simulink model "quadrotorbacksteppingsimulationtracker"  (R2015a)
settings: Solver=ode45  StartTime=0.0  StopTime=15  FixedStep=1e-3  RelTol=1e-3
settings Model: Creator=kbmaj  LastModifiedBy=kbmaj

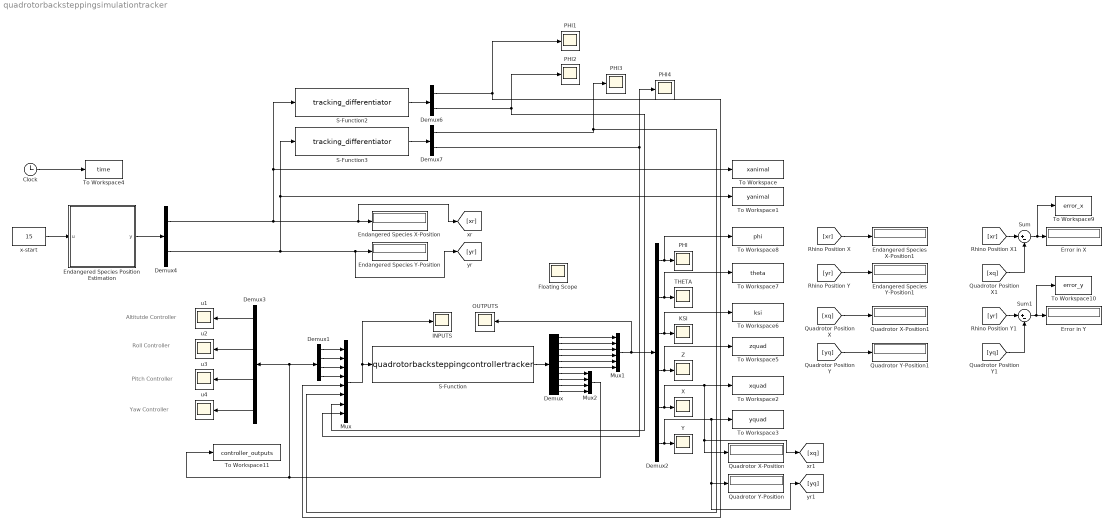
== system quadrotorbacksteppingsimulationtracker ==
  note: Yaw Controller
  note: Pitch Controller
  note: Roll Controller
  note: Altitutde Controller
  Clock : Clock
  Demux : Demux  Outputs=10
  Demux1 : Demux
  Demux2 : Demux  Outputs=6
  Demux3 : Demux
  Demux4 : Demux  Outputs=2
  Demux6 : Demux  Outputs=2
  Demux7 : Demux  Outputs=2
  Endangered Species Position Estimation : MATLAB Function  TreatAsAtomicUnit=on
  Endangered Species X-Position : Display
  Endangered Species X-Position1 : Display
  Endangered Species Y-Position : Display
  Endangered Species Y-Position1 : Display
  Error in X : Display
  Error in Y : Display
  Floating Scope : Scope
      settings: Floating=on  YMin=-30  YMax=45  SaveName=ScopeData12
  INPUTS : Scope
      settings: YMin=-10000  YMax=150000
  KSI : Scope
      settings: YMin=-1359.25  YMax=-1354.25  SaveName=ScopeData4
  Mux : Mux  Inputs=8
  Mux1 : Mux  Inputs=6
  Mux2 : Mux
  OUTPUTS : Scope
      settings: YMin=-10000  YMax=150000  SaveName=ScopeData11
  PHI{,1..4} (5 alike) : Scope
      PHI settings: TimeRange=10  YMin=1250  YMax=3750  SaveName=ScopeData2
      PHI1 settings: TimeRange=10  YMin=9.75  YMax=12.75  SaveName=ScopeData13
      PHI2 settings: TimeRange=10  YMin=1250  YMax=3750  SaveName=ScopeData14
      PHI3 settings: TimeRange=10  YMin=1250  YMax=3750  SaveName=ScopeData15
      PHI4 settings: TimeRange=10  YMin=1250  YMax=3750  SaveName=ScopeData16
  Quadrotor X-Position : Display
  Quadrotor X-Position1 : Display
  Quadrotor Y-Position : Display
  Quadrotor Y-Position1 : Display
  S-Function : S-Function  FunctionName=quadrotorbacksteppingcontrollertracker
  S-Function2 : S-Function  FunctionName=tracking_differentiator
  S-Function3 : S-Function  FunctionName=tracking_differentiator
  Sum : Sum  Inputs=|+-
  Sum1 : Sum  Inputs=|+-
  THETA : Scope
      settings: YMin=19  YMax=21  SaveName=ScopeData3
  To Workspace : ToWorkspace  VariableName=xanimal  SampleTime=-1
  To Workspace1 : ToWorkspace  VariableName=yanimal  SampleTime=-1
  To Workspace10 : ToWorkspace  VariableName=error_y  SampleTime=-1
  To Workspace11 : ToWorkspace  VariableName=controller_outputs  SampleTime=-1
  To Workspace2 : ToWorkspace  VariableName=xquad  SampleTime=-1
  To Workspace3 : ToWorkspace  VariableName=yquad  SampleTime=-1
  To Workspace4 : ToWorkspace  VariableName=time  SampleTime=-1
  To Workspace5 : ToWorkspace  VariableName=zquad  SampleTime=-1
  To Workspace6 : ToWorkspace  VariableName=ksi  SampleTime=-1
  To Workspace7 : ToWorkspace  VariableName=theta  SampleTime=-1
  To Workspace8 : ToWorkspace  VariableName=phi  SampleTime=-1
  To Workspace9 : ToWorkspace  VariableName=error_x  SampleTime=-1
  X : Scope
      settings: TimeRange=5  YMin=7.05  YMax=7.6  SaveName=ScopeData6
  Y : Scope
      settings: YMin=-60  YMax=60  SaveName=ScopeData7
  Z : Scope
      settings: YMin=9350  YMax=9465  SaveName=ScopeData5
  u{1..4} (4 alike) : Scope
      u1 settings: YMin=0  YMax=120000  SaveName=ScopeData8
      u2 settings: TimeRange=25  YMin=-0.2  YMax=0.5
      u3 settings: YMin=0  YMax=120000  SaveName=ScopeData10
      u4 settings: YMin=0  YMax=120000  SaveName=ScopeData9
  x-start : Constant  Value=15
  wires:
  S-Function/1 -> Demux/1
  Mux/1 -> INPUTS/1, S-Function/1
  Demux/1 -> Mux1/1
  Demux/2 -> Mux1/2
  Demux/3 -> Mux1/3
  Demux/4 -> Mux1/4
  Demux/5 -> Mux1/5
  Demux/6 -> Mux1/6
  Mux1/1 -> OUTPUTS/1, Demux2/1
  Demux2/1 -> To Workspace8/1, PHI/1
  Demux2/2 -> To Workspace7/1, THETA/1
  Demux2/3 -> To Workspace6/1, KSI/1
  Demux2/4 -> To Workspace5/1, Z/1
  Demux2/5 -> To Workspace2/1, [xq], Quadrotor X-Position/1, X/1
  Demux/7 -> Mux2/1
  Demux/8 -> Mux2/2
  Demux/9 -> Mux2/3
  Demux/10 -> Mux2/4
  Demux1/1 -> Mux/1
  Demux1/2 -> Mux/2
  Demux1/3 -> Mux/3
  Demux1/4 -> Mux/4
  Mux2/1 -> Demux1/1, Demux3/1, To Workspace11/1
  Demux3/1 -> u1/1
  Demux3/2 -> u2/1
  Demux3/3 -> u3/1
  Demux3/4 -> u4/1
  x-start/1 -> Endangered Species Position Estimation/1(u)
  Demux4/1 -> [xr], Endangered Species X-Position/1, S-Function2/1, To Workspace/1
  Demux4/2 -> [yr], Endangered Species Y-Position/1, S-Function3/1, To Workspace1/1
  Demux2/6 -> To Workspace3/1, [yq], Quadrotor Y-Position/1, Y/1
  Clock/1 -> To Workspace4/1
  Endangered Species Position Estimation/1(y) -> Demux4/1
  [xr] -> Endangered Species X-Position1/1
  [yr] -> Endangered Species Y-Position1/1
  [xq] -> Quadrotor X-Position1/1
  [yq] -> Quadrotor Y-Position1/1
  [xr] -> Sum/1
  [xq] -> Sum/2
  [yr] -> Sum1/1
  [yq] -> Sum1/2
  Sum1/1 -> To Workspace10/1, Error in Y/1
  Sum/1 -> To Workspace9/1, Error in X/1
  Demux6/1 -> Mux/5, PHI1/1
  Demux6/2 -> Mux/7, PHI2/1
  Demux7/1 -> PHI3/1, Mux/6
  Demux7/2 -> PHI4/1, Mux/8
  S-Function2/1 -> Demux6/1
  S-Function3/1 -> Demux7/1

== matlab function quadrotorbacksteppingsimulationtracker/Endangered Species Position Estimation ==
  data: y output; u input
function y = tracker(u)
%#codegen

% Initialization
B       = 1;  % distance between wheels
dt      = 1;  % sampling time
X       = 0;  % x-position of sensor
Y       = 0;  % y-position of sensor
v       = 1.5;        % velocity
%varphi  = 2.5*pi/80; % steering angle

% Noise Signals - q(k),r(k)
% Process(Q) and Observation(R) noise varainces, mean 0
mu          = 0;
sigma_x     = 0.05;
sigma_y     = 0.05;
sigma_phi   = pi/180;
sigma_r     = 0.5;
sigma_theta = 2*pi/180;

Q           = diag([sigma_x, sigma_y, sigma_phi].^2);
R           = diag([sigma_r, sigma_theta].^2);
p           = diag([0.0001 0.0001 0.000001]);

% System Initial States
x       = [ u ; -22; 0];
x_hat   = [ 15; -23; 0];

% Instance
kk = 50;
% Preallocation
 xestpos     = zeros(kk,1)';
 yestpos     = zeros(kk,1)';
% Discrete Dynamic Model

for k = 1:kk
% System Noises
qn          = [sigma_x*randn(1)+mu;  sigma_y*randn(1)+mu;  sigma_phi*randn(1)+mu]; % process noise
rn          = [sigma_r*randn(1)+mu;  sigma_theta*randn(1)+mu]; % measurement noise

% if k > 0 && k < 23
%         varphi  = 2.5*pi/80;
%     elseif k > 23 && k < 28
%         varphi = 0;
%     else if k >28 && k < 50
%         varphi = -2.5*pi/100;
%     end
% end

if k > 0 && k < 25;
varphi  =  2.5*pi/80;
else k > 25 && k <60;
varphi  = -2.5*pi/80;
end

% Model
% Perfect System Model - x(k+1)
x  =   x + [dt* v* cos(x(3)+varphi);
            dt* v* sin(x(3)+varphi);
            dt* (v/B) *(sin(varphi))];
x = x + qn;
% Perfect Output measurement
z    =       [sqrt((X-x(1))^2 + (Y-x(2))^2);
            atan(((Y-(x(2)))/(X-(x(1))))-((x(3))))];
Z = z + rn;
% EKF Model and Measurement
x_hat  = x_hat +  [dt* v* cos(x_hat(3)+varphi);
                   dt* v* sin(x_hat(3)+varphi);
                   dt* (v/B)*(sin(varphi))];
% Z measurement
Zh   = [sqrt((X-(x_hat(1)))^2 + (Y-x_hat(2))^2 );
       atan(((Y-(x_hat(2)))/((X-(x_hat(1)))))-((x_hat(3))))];

% F Model Jacobian
F_jac     =  [1 0  -dt*v*sin(x_hat(3) + varphi)
              0 1   dt*v*cos(x_hat(3) + varphi)
              0 0   1                         ];
% H Measurement Jacobian
d       = sqrt((X-x_hat(1))^2+(Y-x_hat(2))^2);
H_jac   = [(x_hat(1)-X)/d    (x_hat(2)-Y)/d      0
          -(x_hat(2)-Y)/d^2  (x_hat(1)-X)/d^2   -1];

% Prediction Function
p   =  F_jac * p * F_jac' + Q;

% Updates
S   =  H_jac * p       * H_jac' + R;
K   =  p     * H_jac'  * inv(S);

% Estimates
x_est = x_hat + K*(Z-Zh);
p_est = p - K*S*K';
%x_est;

xestpos(k) = x_est(1);
yestpos(k) = x_est(2);
xxx = x_est(1);
yyy = x_est(2);
end



y = [xxx ; yyy];
